simulink model "zuijia"  (R2016b)
settings: Solver=VariableStepAuto  StartTime=0.0  StopTime=10.0  RelTol=1e-3
settings Model: Creator=white  LastModifiedBy=white

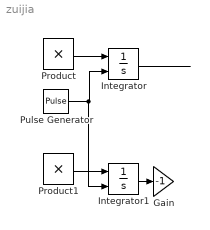
== system zuijia ==
  Gain : Gain  Gain=-1
  Integrator : Integrator  ExternalReset=rising
  Integrator1 : Integrator  ExternalReset=rising
  Product : Product
  Product1 : Product
  Pulse Generator : DiscretePulseGenerator  PulseType=Time based  Period=1/800  PulseWidth=5
  wires:
  Product/1 -> Integrator/1
  Product1/1 -> Integrator1/1
  Integrator/1 -> ?
  Integrator1/1 -> Gain/1
  Pulse Generator/1 -> Integrator1/2, Integrator/2
